simulink model "TX_TUNE_DIGITALv5"  (R2024a)
settings: Solver=VariableStepAuto  StartTime=0.0  StopTime=0.15e-3  FixedStep=1e-9  RelTol=1e-3
values from neighbouring files (symbols this model uses):
  cnt_min = 10    [TX_PM_MODEL_Setup.m]
  fin = 1e6    (= 1000000)    [TX_PM_MODEL_Setup.m]
  tcmp = 5    [TX_PM_MODEL_Setup.m]
libraries: MyLibTwoSwitchConfig x4, dspsigops x2, simulink x1
settings Model: Creator=cian.odonnell  LastModifiedBy=ciano
settings SolverCC: EnableFixedStepZeroCrossing=on

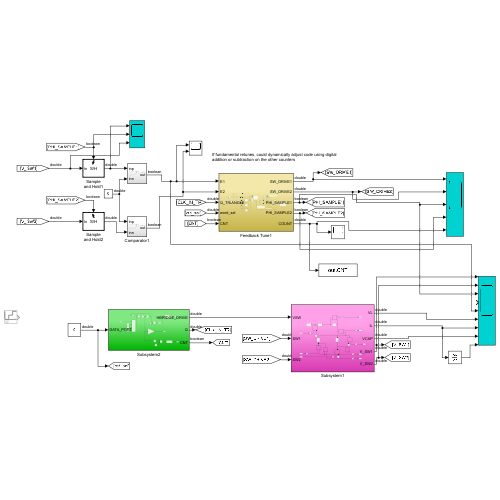
[thumbnail: Simulink's stored preview of the top-level diagram]
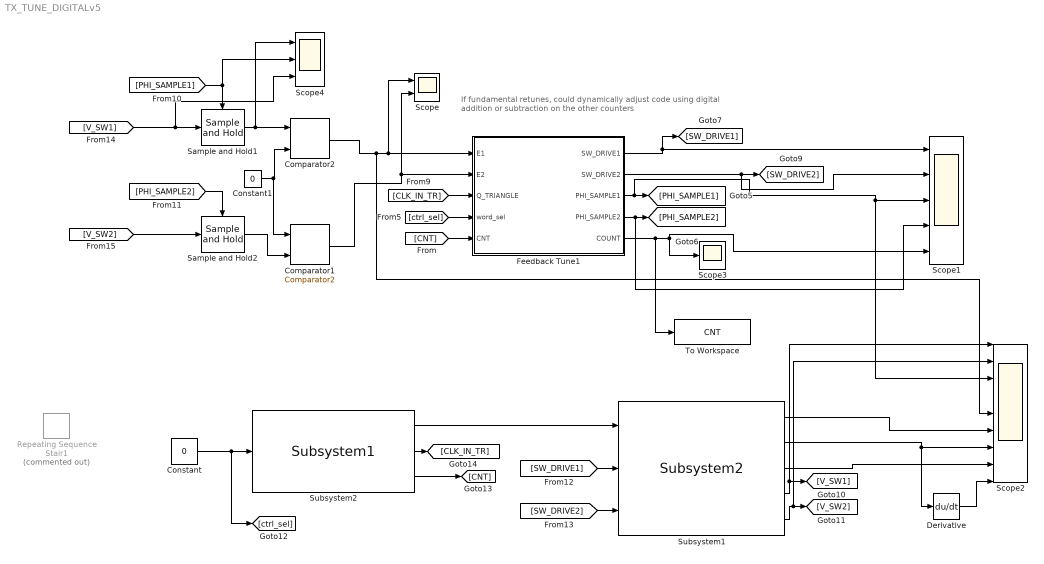
== system TX_TUNE_DIGITALv5 ==
  note: If fundamental retunes, could dynamically adjust code using digital
      | addition or subtraction on the other counters
  Comparator1 : MyLibTwoSwitchConfig/Comparator2  SystemSampleTime=-1  VariantActivationTime=update diagram  AllowFlexibleInterface=on  Latency=0  AutoFrameSizeCalculation=off
  Comparator2 : MyLibTwoSwitchConfig/Comparator2  SystemSampleTime=-1  VariantActivationTime=update diagram  AllowFlexibleInterface=on  Latency=0  AutoFrameSizeCalculation=off
  Constant : Constant  Value=0
  Constant1 : Constant  Value=0
  Derivative : Derivative
  Feedback Tune1 : Subsystem
  Repeating Sequence Stair1 : simulink/Sources/Repeating Sequence Stair  Commented=on  OutValues=[0 1 2].'  tsamp=20/fin  OutMin=[]  OutMax=[]  OutDataTypeStr=double  OutputDataTypeScalingMode=double  OutDataType=fixdt(0,8)  ConRadixGroup=Best Precision: Vector-wise  OutScaling=2^-12
  Sample and Hold1 : dspsigops/Sample and Hold  trig=Rising edge  initCond=0  latchinput=off
  Sample and Hold2 : dspsigops/Sample and Hold  trig=Falling edge  initCond=0  latchinput=off
  Scope : Scope  NumInputPorts=2
  Scope1 : Scope  NumInputPorts=5
  Scope2 : Scope  NumInputPorts=9
  Scope3 : Scope
  Scope4 : Scope  NumInputPorts=3
  Subsystem1 : MyLibTwoSwitchConfig/Subsystem2  SystemSampleTime=-1  VariantActivationTime=update diagram  AllowFlexibleInterface=on  Latency=0  AutoFrameSizeCalculation=off
  Subsystem2 : MyLibTwoSwitchConfig/Subsystem1  SystemSampleTime=-1  VariantActivationTime=update diagram  AllowFlexibleInterface=on  Latency=0  AutoFrameSizeCalculation=off
  To Workspace : ToWorkspace  VariableName=CNT  SaveFormat=Timeseries  SampleTime=-1
      settings: MaxDataPoints=1  Save2DSignal=2-D array (concatenate along first dimension)
  wires:
  [ctrl_sel] -> Feedback Tune1/4(word_sel)
  [CLK_IN_TR] -> Feedback Tune1/3(Q_TRIANGLE)
  Feedback Tune1/2(SW_DRIVE2) -> Scope1/2, [SW_DRIVE2]
  Feedback Tune1/1(SW_DRIVE1) -> Scope1/1, [SW_DRIVE1]
  Feedback Tune1/3(PHI_SAMPLE1) -> Scope2/3, Scope1/3, [PHI_SAMPLE1]
  Feedback Tune1/4(PHI_SAMPLE2) -> Scope1/4, [PHI_SAMPLE2]
  Feedback Tune1/5(COUNT) -> Scope3/1, Scope1/5, To Workspace/1
  Constant1/1 -> Comparator1/1, Comparator2/2
  [PHI_SAMPLE1] -> Scope4/2, Sample and Hold1/Trigger
  [PHI_SAMPLE2] -> Sample and Hold2/Trigger
  Subsystem1/4 -> Scope2/1, [V_SW1]
  Subsystem1/5 -> Scope2/2, [V_SW2]
  [SW_DRIVE1] -> Subsystem1/2
  [SW_DRIVE2] -> Subsystem1/3
  Subsystem2/1 -> Subsystem1/1
  Constant/1 -> Subsystem2/1, [ctrl_sel]
  Subsystem2/2 -> [CLK_IN_TR]
  Subsystem2/3 -> [CNT]
  Sample and Hold1/1 -> Comparator2/1, Scope4/1
  Comparator2/1 -> Scope2/5, Feedback Tune1/1(E1), Scope/1
  Comparator1/1 -> Scope/2, Feedback Tune1/2(E2)
  Subsystem1/1 -> Scope2/6
  Subsystem1/2 -> Derivative/1, Scope2/7
  Subsystem1/3 -> Scope2/8
  [V_SW2] -> Sample and Hold2/1
  [V_SW1] -> Scope4/3, Sample and Hold1/1
  Sample and Hold2/1 -> Comparator1/2
  [CNT] -> Feedback Tune1/5(CNT)
  Derivative/1 -> Scope2/9

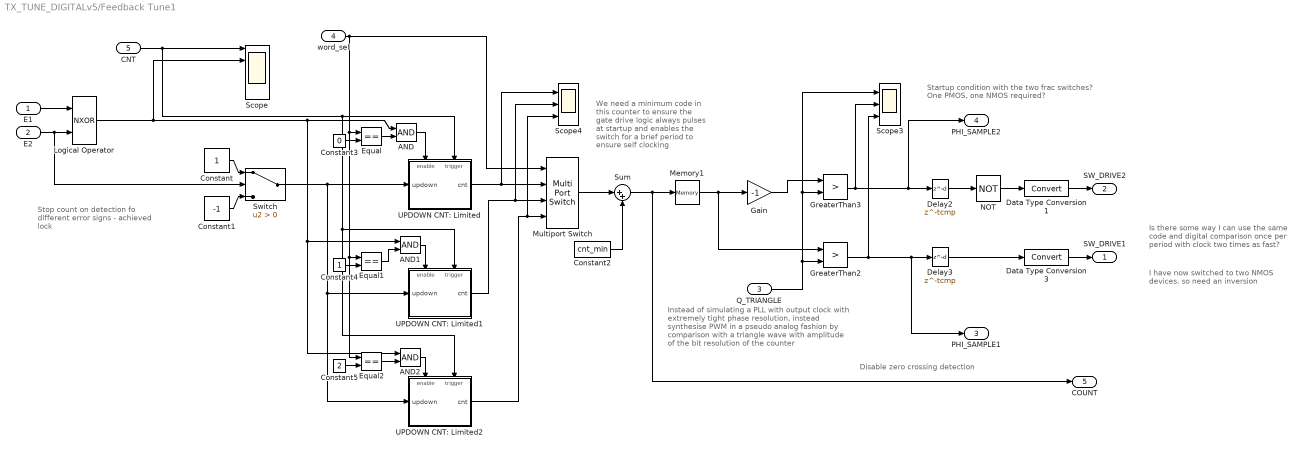
== system TX_TUNE_DIGITALv5/Feedback Tune1 ==
  note: I have now switched to two NMOS devices. so need an inversion
  note: Startup condition with the two frac switches?
      | One PMOS, one NMOS required?
  note: Stop count on detection fo different error signs - achieved lock
  note: Instead of simulating a PLL with output clock with extremely tight phase resolution, instead synthesise PWM in a pseudo analog fashion by comparison with a triangle wave with amplitude of the bit resolution of the counter
  note: Disable zero crossing detection
  note: We need a minimum code in this counter to ensure the gate drive logic always pulses at startup and enables the switch for a brief period to ensure self clocking
  note: Is there some way I can use the same code and digital comparison once per period with clock two times as fast?
  E1 : Inport
  E2 : Inport  Port=2
  Q_TRIANGLE : Inport  Port=3
  word_sel : Inport  Port=4
  CNT : Inport  Port=5
  AND : Logic  IconShape=distinctive  AllPortsSameDT=off  OutDataTypeStr=boolean
  AND1 : Logic  IconShape=distinctive  AllPortsSameDT=off  OutDataTypeStr=boolean
  AND2 : Logic  IconShape=distinctive  AllPortsSameDT=off  OutDataTypeStr=boolean
  Constant : Constant
  Constant1 : Constant  Value=-1
  Constant2 : Constant  Value=cnt_min
  Constant3 : Constant  Value=0
  Constant4 : Constant
  Constant5 : Constant  Value=2
  Data Type Conversion1 : DataTypeConversion  SaturateOnIntegerOverflow=off  RndMeth=Floor
  Data Type Conversion3 : DataTypeConversion  SaturateOnIntegerOverflow=off  RndMeth=Floor
  Delay2 : Delay  DelayLength=tcmp  SampleTime=1e-9
  Delay3 : Delay  DelayLength=tcmp  SampleTime=1e-9
  Equal : RelationalOperator  Operator===  OutDataTypeStr=boolean  RndMeth=Simplest  InputSameDT=off
  Equal1 : RelationalOperator  Operator===  OutDataTypeStr=boolean  RndMeth=Simplest  InputSameDT=off
  Equal2 : RelationalOperator  Operator===  OutDataTypeStr=boolean  RndMeth=Simplest  InputSameDT=off
  Gain : Gain  Gain=-1
  GreaterThan2 : RelationalOperator  Operator=>  OutDataTypeStr=boolean  ZeroCross=off  RndMeth=Simplest  InputSameDT=off
  GreaterThan3 : RelationalOperator  Operator=>  OutDataTypeStr=boolean  ZeroCross=off  RndMeth=Simplest  InputSameDT=off
  Logical Operator : Logic  Operator=NXOR  AllPortsSameDT=off  OutDataTypeStr=boolean
  Memory1 : Memory
  Multiport Switch : MultiPortSwitch  DataPortOrder=Zero-based contiguous  zeroidx=on  SaturateOnIntegerOverflow=off  InputSameDT=off
  NOT : Logic  Operator=NOT  IconShape=distinctive  AllPortsSameDT=off  OutDataTypeStr=boolean
  Scope : Scope  NumInputPorts=5
  Scope3 : Scope  NumInputPorts=3
  Scope4 : Scope  NumInputPorts=3
  Sum : Sum  Inputs=|++
  Switch : Switch  Criteria=u2 > Threshold  ZeroCross=off  SaturateOnIntegerOverflow=off  InputSameDT=off
  UPDOWN CNT: Limited : Subsystem
  UPDOWN CNT: Limited1 : Subsystem
  UPDOWN CNT: Limited2 : Subsystem
  SW_DRIVE1 : Outport
  SW_DRIVE2 : Outport  Port=2
  PHI_SAMPLE1 : Outport  Port=3
  PHI_SAMPLE2 : Outport  Port=4
  COUNT : Outport  Port=5
  wires:
  Memory1/1 -> Gain/1, GreaterThan2/1
  UPDOWN CNT: Limited/1(cnt) -> Scope4/1, Multiport Switch/2
  Switch/1 -> UPDOWN CNT: Limited/1(updown), UPDOWN CNT: Limited2/1(updown), UPDOWN CNT: Limited1/1(updown)
  Constant/1 -> Switch/1
  Constant1/1 -> Switch/3
  Data Type Conversion3/1 -> SW_DRIVE1/1
  Data Type Conversion1/1 -> SW_DRIVE2/1
  Delay3/1 -> Data Type Conversion3/1
  GreaterThan2/1 -> PHI_SAMPLE1/1, Delay3/1, Scope3/3
  Q_TRIANGLE/1 -> GreaterThan3/2, Scope3/1, GreaterThan2/2
  word_sel/1 -> Equal2/1, Equal1/1, Equal/1, Multiport Switch/1
  Constant2/1 -> Sum/2
  Multiport Switch/1 -> Sum/1
  Sum/1 -> COUNT/1, Memory1/1
  CNT/1 -> UPDOWN CNT: Limited/Trigger, UPDOWN CNT: Limited2/Trigger, UPDOWN CNT: Limited1/Trigger, Scope/1
  UPDOWN CNT: Limited1/1(cnt) -> Scope4/2, Multiport Switch/3
  UPDOWN CNT: Limited2/1(cnt) -> Scope4/3, Multiport Switch/4
  Constant3/1 -> Equal/2
  Constant4/1 -> Equal1/2
  Constant5/1 -> Equal2/2
  E2/1 -> Switch/2, Logical Operator/2
  Logical Operator/1 -> AND/1, AND2/1, AND1/1, Scope/2
  AND/1 -> UPDOWN CNT: Limited/Enable
  Equal/1 -> AND/2
  AND1/1 -> UPDOWN CNT: Limited1/Enable
  Equal1/1 -> AND1/2
  AND2/1 -> UPDOWN CNT: Limited2/Enable
  Equal2/1 -> AND2/2
  E1/1 -> Logical Operator/1
  Delay2/1 -> NOT/1
  GreaterThan3/1 -> PHI_SAMPLE2/1, Delay2/1, Scope3/2
  Gain/1 -> GreaterThan3/1
  NOT/1 -> Data Type Conversion1/1

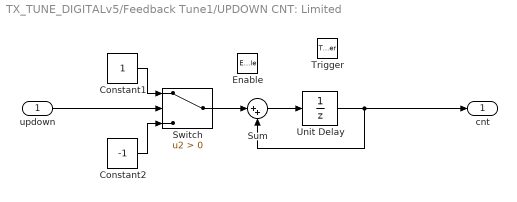
== system TX_TUNE_DIGITALv5/Feedback Tune1/UPDOWN CNT: Limited ==
  updown : Inport
  Enable : EnablePort
  Trigger : TriggerPort  TriggerType=either  VariantControl=(inherit)  PortDimensions=1
  Constant1 : Constant
  Constant2 : Constant  Value=-1
  Sum : Sum  Inputs=|++
  Switch : Switch  Criteria=u2 > Threshold  SaturateOnIntegerOverflow=off  InputSameDT=off
  Unit Delay : UnitDelay  SampleTime=-1  HasFrameUpgradeWarning=on
  cnt : Outport
  wires:
  Switch/1 -> Sum/1
  Constant2/1 -> Switch/3
  Sum/1 -> Unit Delay/1
  updown/1 -> Switch/2
  Constant1/1 -> Switch/1
  Unit Delay/1 -> cnt/1, Sum/2

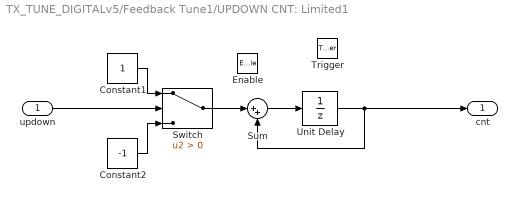
== system TX_TUNE_DIGITALv5/Feedback Tune1/UPDOWN CNT: Limited1 ==
  updown : Inport
  Enable : EnablePort
  Trigger : TriggerPort  TriggerType=either  VariantControl=(inherit)  PortDimensions=1
  Constant1 : Constant
  Constant2 : Constant  Value=-1
  Sum : Sum  Inputs=|++
  Switch : Switch  Criteria=u2 > Threshold  SaturateOnIntegerOverflow=off  InputSameDT=off
  Unit Delay : UnitDelay  SampleTime=-1  HasFrameUpgradeWarning=on
  cnt : Outport
  wires:
  Switch/1 -> Sum/1
  Constant2/1 -> Switch/3
  Sum/1 -> Unit Delay/1
  updown/1 -> Switch/2
  Constant1/1 -> Switch/1
  Unit Delay/1 -> cnt/1, Sum/2

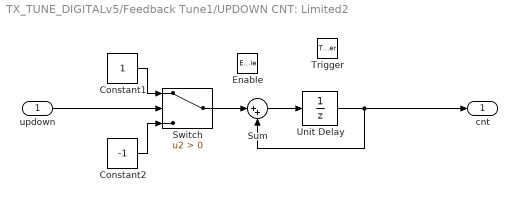
== system TX_TUNE_DIGITALv5/Feedback Tune1/UPDOWN CNT: Limited2 ==
  updown : Inport
  Enable : EnablePort
  Trigger : TriggerPort  TriggerType=either  VariantControl=(inherit)  PortDimensions=1
  Constant1 : Constant
  Constant2 : Constant  Value=-1
  Sum : Sum  Inputs=|++
  Switch : Switch  Criteria=u2 > Threshold  SaturateOnIntegerOverflow=off  InputSameDT=off
  Unit Delay : UnitDelay  SampleTime=-1  HasFrameUpgradeWarning=on
  cnt : Outport
  wires:
  Switch/1 -> Sum/1
  Constant2/1 -> Switch/3
  Sum/1 -> Unit Delay/1
  updown/1 -> Switch/2
  Constant1/1 -> Switch/1
  Unit Delay/1 -> cnt/1, Sum/2
